simulink model "PC_Quadcopter_Simulation_BackStepping_ISE"  (R2015b)
settings: Solver=FixedStepAuto  StartTime=0.0  StopTime=10  FixedStep=0.02  RelTol=1e-3
settings Model: Creator=HKJ  LastModifiedBy=HL

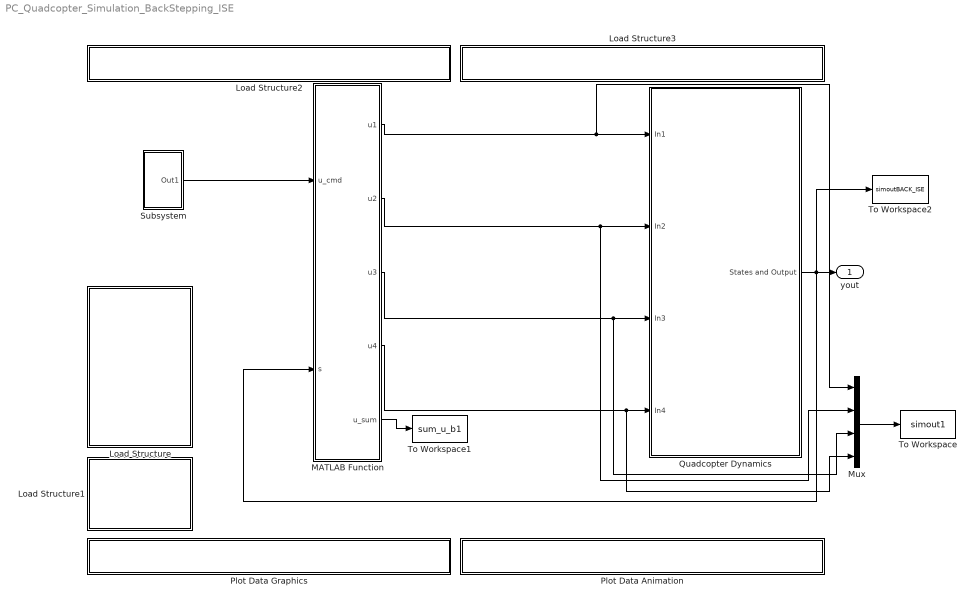
== system PC_Quadcopter_Simulation_BackStepping_ISE ==
  Load Structure : Subsystem
      settings: OpenFcn=|
      | uiopen('load')
      | if (exist('IC')==1 && exist('quadModel')==1)
      | set_param(bdroot, 'SimulationCommand', 'update')
      | end
      mask Display: fprintf('LOAD:\nQuadcopter\nModel Or\nInitial\nConditions');
  Load Structure1 : Subsystem
      settings: OpenFcn=|
      | if (exist('IC')==1 && exist('quadModel')==1 && exist('yout') && exist('tout'))
      | saveSimResults()
      | else
      | msgbox('No Data To Save!')
      | end
      mask Display: fprintf('SAVE:\nSimulation\nResults');
  Load Structure2 : Subsystem
      settings: OpenFcn=|
      | if exist('GUI_Modeling') == 2,
      | run('GUI_Modeling')
      | 
      | else
      | 
      | msgbox('The desired GUI must be first added to MATLABs path.')
      | 
      | end
      mask Display: fprintf('OPEN GUI: Build New \n Model');
  Load Structure3 : Subsystem
      settings: OpenFcn=|
      | if exist('GUI_IC') == 2,
      | run('GUI_IC')
      | 
      | else
      | 
      | msgbox('The desired GUI must be first added to MATLABs path.')
      | 
      | end
      mask Display: fprintf('OPEN GUI: Create Initial \n Conditions');
  MATLAB Function : MATLAB Function  TreatAsAtomicUnit=on
  Mux : Mux
  Plot Data Animation : Subsystem
      settings: OpenFcn=|
      | if exist('QuadAnim4') == 2,
      |     if exist('yout')
      | 	run('QuadAnim4');
      |     else
      |     msgbox('Simulation must be run before data can be plotted.');
      |     end
      | else                                                                          msgbox('The desired GUI must be first added to MATLABs path.')
      | end
      mask Display: fprintf('OPEN GUI: Flight Animation')
  Plot Data Graphics : Subsystem
      settings: OpenFcn=|
      | if exist('yout')
      | yout = evalin('base', 'yout');
      | tout = evalin('base', 'tout');
      | quadPlots(yout, tout)
      | else
      | msgbox('Simulation must be run before data can be plotted.')
      | end
      mask Display: fprintf('OPEN PLOT: State Data')
  Quadcopter Dynamics : Subsystem
  Subsystem : Subsystem
  To Workspace : ToWorkspace  VariableName=simout1  SampleTime=-1
      settings: Save2DSignal=2-D array (concatenate along first dimension)
  To Workspace1 : ToWorkspace  VariableName=sum_u_b1  SampleTime=-1
      settings: Save2DSignal=2-D array (concatenate along first dimension)
  To Workspace2 : ToWorkspace  VariableName=simoutBACK_ISE  SampleTime=-1
      settings: Save2DSignal=2-D array (concatenate along first dimension)
  yout : Outport
  wires:
  Quadcopter Dynamics/1(States and Output) -> To Workspace2/1, MATLAB Function/2(s), yout/1
  MATLAB Function/1(u1) -> Mux/1, Quadcopter Dynamics/1(In1)
  MATLAB Function/2(u2) -> Mux/2, Quadcopter Dynamics/2(In2)
  MATLAB Function/3(u3) -> Mux/3, Quadcopter Dynamics/3(In3)
  MATLAB Function/4(u4) -> Mux/4, Quadcopter Dynamics/4(In4)
  Subsystem/1(Out1) -> MATLAB Function/1(u_cmd)
  Mux/1 -> To Workspace/1
  MATLAB Function/5(u_sum) -> To Workspace1/1

== system PC_Quadcopter_Simulation_BackStepping_ISE/Load Structure ==

== system PC_Quadcopter_Simulation_BackStepping_ISE/Load Structure1 ==

== system PC_Quadcopter_Simulation_BackStepping_ISE/Load Structure2 ==

== system PC_Quadcopter_Simulation_BackStepping_ISE/Load Structure3 ==

== system PC_Quadcopter_Simulation_BackStepping_ISE/Plot Data Animation ==

== system PC_Quadcopter_Simulation_BackStepping_ISE/Plot Data Graphics ==

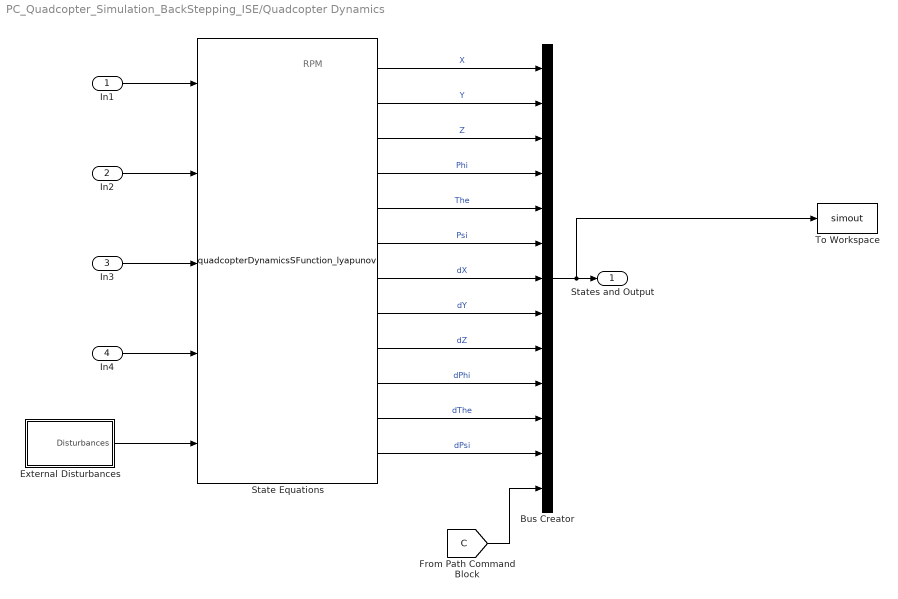
== system PC_Quadcopter_Simulation_BackStepping_ISE/Quadcopter Dynamics ==
  note: RPM
  In1 : Inport
  In2 : Inport  Port=2
  In3 : Inport  Port=3
  In4 : Inport  Port=4
  Bus Creator : BusCreator  Inputs='X','Y','Z','Phi','The','Psi','dX','dY','dZ','dPhi','dThe','dPsi','XY_Cmd'
  External Disturbances : Subsystem
  State Equations : M-S-Function  FunctionName=quadcopterDynamicsSFunction_lyapunov  Parameters=quadModel, IC
      mask Display:
      | port_label('input', 1, 'RPM1')
      | port_label('input', 2, 'RPM2')
      | port_label('input', 3, 'RPM3')
      | port_label('input', 4, 'RPM4')
      | port_label('input', 5, 'Disturbances')
      | port_label('output', 1, 'X')
      | port_label('output', 2, 'Y')
      | port_label('output', 3, 'Z')
      | port_label('output', 4, 'Phi')
      | port_label('output', 5, 'The')
      | port_label('output', 6, 'Psi')
      | port_label('output', 7, 'dX')
      | port_label('output', 8, 'dY')
      | port_label('output', 9, 'dZ')
      | port_label('output', 10, 'dPhi')
      | port_label('output', 11, 'dThe')
      | port_label('output', 12, 'dPsi')
  To Workspace : ToWorkspace  VariableName=simout  SampleTime=-1
      settings: Save2DSignal=2-D array (concatenate along first dimension)
  States and Output : Outport
  wires:
  [C] -> Bus Creator/13
  External Disturbances/1("Disturbances ") -> State Equations/5
  Bus Creator/1 -> To Workspace/1, States and Output/1
  State Equations/12 -> Bus Creator/12  "dPsi"
  State Equations/11 -> Bus Creator/11  "dThe"
  State Equations/10 -> Bus Creator/10  "dPhi"
  State Equations/9 -> Bus Creator/9  "dZ"
  State Equations/8 -> Bus Creator/8  "dY"
  State Equations/7 -> Bus Creator/7  "dX"
  State Equations/6 -> Bus Creator/6  "Psi"
  State Equations/5 -> Bus Creator/5  "The"
  State Equations/4 -> Bus Creator/4  "Phi"
  State Equations/3 -> Bus Creator/3  "Z"
  State Equations/2 -> Bus Creator/2  "Y"
  State Equations/1 -> Bus Creator/1  "X"
  In4/1 -> State Equations/4
  In3/1 -> State Equations/3
  In2/1 -> State Equations/2
  In1/1 -> State Equations/1

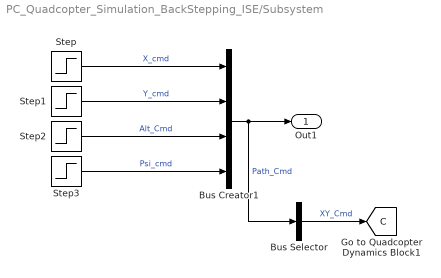
== system PC_Quadcopter_Simulation_BackStepping_ISE/Subsystem ==
  Bus Creator1 : BusCreator  Inputs=4
  Bus Selector : BusSelector  OutputSignals=X_cmd,Y_cmd  OutputAsBus=on
  Step : Step  Time=0
  Step1 : Step  Time=0
  Step2 : Step  Time=0  After=-1
  Step3 : Step  Time=0  After=0
  Out1 : Outport
  tag scope: C=global
  wires:
  Step3/1 -> Bus Creator1/4  "Psi_cmd"
  Step2/1 -> Bus Creator1/3  "Alt_Cmd"
  Step/1 -> Bus Creator1/1  "X_cmd"
  Step1/1 -> Bus Creator1/2  "Y_cmd"
  Bus Creator1/1 -> Bus Selector/1, Out1/1  "Path_Cmd"
  Bus Selector/1 -> [C]  "XY_Cmd"

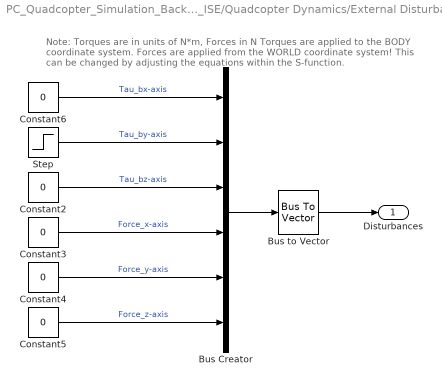
== system PC_Quadcopter_Simulation_BackStepping_ISE/Quadcopter Dynamics/External Disturbances ==
  note: Note: Torques are in units of N*m, Forces in N
      | Torques are applied to the BODY coordinate system.
      | Forces are applied from the WORLD coordinate system!
      | This can be changed by adjusting the equations within the S-function.
  Bus Creator : BusCreator  Inputs=6
  Bus to Vector : BusToVector
  Constant{2..6} (5 alike) : Constant  Value=0
  Step : Step  After=0  SampleTime=0
  "Disturbances " : Outport
  wires:
  Constant5/1 -> Bus Creator/6  "Force_z-axis"
  Constant4/1 -> Bus Creator/5  "Force_y-axis"
  Constant3/1 -> Bus Creator/4  "Force_x-axis"
  Constant2/1 -> Bus Creator/3  "Tau_bz-axis"
  Step/1 -> Bus Creator/2  "Tau_by-axis"
  Constant6/1 -> Bus Creator/1  "Tau_bx-axis"
  Bus Creator/1 -> Bus to Vector/1
  Bus to Vector/1 -> "Disturbances "/1

== matlab function PC_Quadcopter_Simulation_BackStepping_ISE/MATLAB Function ==
  data: u_cmd input; u1 output; s input; u2 output; u3 output; u4 output; u_sum output
function [u1,u2,u3,u4,u_sum] = fcn(u_cmd,s)
k1 = 3;
k2 = 3;
k3 = 3;
k4 = 3;
k5 = 2.2;
k6 = 2.2;
k7= 0.466;
k8= 3;
k9= 0.466;
k10= 3;
k11= 0.3;
k12= 3;

Ix = 0.0094999;Iy=0.0094999;Iz=0.018576;
m=1.023;g=9.81;
L=0.185738;

x_cmd = u_cmd(1);
y_cmd = u_cmd(2);
alt_cmd = u_cmd(3);
psi_cmd = u_cmd(4);
x = s(1);y = s(2);z = s(3);
phi = s(4);the = s(5);psi = s(6);
dx = s(7);dy = s(8);dz = s(9);
dphi = s(10);dthe = s(11);dpsi = s(12);

e7 = z-alt_cmd;
e8 = dz + k7*e7;
e9 = x - x_cmd;
e10 = dx + k9*e9;
e11 = y - y_cmd;
e12 = dy + k11*e11;

u1 = m*(g+(k7^2-1)*e7-(k7+k8)*e8)/(cos(phi)*cos(the));
% r1 = -Limit(e10, -5, 5)/5*1;
% r2 = -Limit(e12, -5, 5)/5*1;
r1 = m/u1*(-(k9+k10)*e10+(k9^2-1)*e9);
r2 = m/u1*(-(k11+k12)*e12+(k11^2-1)*e11);
phi_cmd = asin(r1*sin(psi)-r2*cos(psi));
the_cmd = asin((r1*cos(psi)+r2*sin(psi))/cos(phi_cmd));


e1 = phi-phi_cmd;
e2 = dphi+k1*e1;
e3 = the-the_cmd;
e4 = dthe+k3*e3;
e5 = psi-psi_cmd;
e6 = dpsi+k5*e5;

u2 =Ix/L*(-dthe*dpsi*(Iy-Iz)/Ix+(k1^2-1)*e1-(k1+k2)*e2);
u3 =Iy/L*(-dphi*dpsi*(Iz-Ix)/Iy+(k3^2-1)*e3-(k3+k4)*e4);
u4 =Iz*(-dthe*dphi*(Ix-Iy)/Iz+(k5^2-1)*e5-(k5+k6)*e6);

u_sum = u1*u1+u2*u2+u3*u3+u4*u4;
